simulink model "Peltier_OpenLoop_Simulink_Controller"  (R2018a)
settings: Solver=ode3  StartTime=0.0  StopTime=100  FixedStep=1/1000  RelTol=1e-3  EnableMultiTasking=on
libraries: simulink x1
settings Model: Creator=g.reynosomeza  LastModifiedBy=Pichau
settings DataIOCC: LimitDataPoints=on  SaveFormat=Array
settings OptimizationCC: LifeSpan=inf
settings DebuggingCC: AlgebraicLoopMsg=none  ArtificialAlgebraicLoopMsg=none  SolverPrmCheckMsg=warning  SFUnexpectedBacktrackingDiag=warning  SFNoUnconditionalDefaultTransitionDiag=warning  SFExecutionAtInitializationDiag=none
settings HardwareCC: ProdBitPerPointer=32  ProdBitPerSizeT=32  ProdBitPerPtrDiffT=32  ProdLargestAtomicFloat=None  ProdIntDivRoundTo=Undefined  ProdEndianess=Unspecified  ProdWordSize=32  ProdHWDeviceType=32-bit Generic
settings ModelReferenceCC: PropagateSignalLabelsOutOfModel=off
settings CodeAppCC: StateflowObjectComments=on
settings GRTTargetCC: TargetLangStandard=C89/C90 (ANSI)  GeneratePreprocessorConditionals=Disable all
settings ConfigComp: CovMetricSettings=dw  CovHtmlReporting=on  CovSaveCumulativeToWorkspaceVar=on  CovSaveSingleToWorkspaceVar=on  CovExternalEMLEnable=off  CovSFcnEnable=off

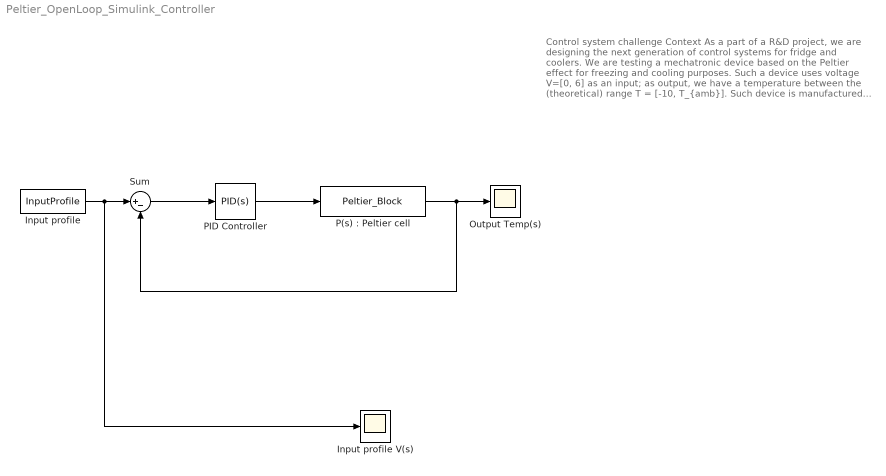
== system Peltier_OpenLoop_Simulink_Controller ==
  note: Control system challenge
      |
      | Context
      |
      | As a part of a R&D project, we are designing the next generation
      | of control systems for fridge and coolers. We are testing a mechatronic
      | device based on the Peltier effect for freezing and cooling purposes.
      | Such a device uses voltage V=[0, 6] as an input; as output, we have a
      | temperature between the (theoretical) range T = [-10, T_{amb}].
      |
      | Such device is manufactured in mass, and therefore, some differences
      | regarding physical properties are expected. We have a preliminary step-test
      | in order to appreciate the non-linear dynamic of the process.
      |
      | Task to perform
      |
      | It is desired to tune a controller, for the nominal process and robust enough
      | to handle the expected differences in its physical properties.
      |
      | 1) Controller performance will be evaluated with the IAE and TV indexes.
      | 2) Such controller must have a better performance when compared with a
      | controller adjusted with the Ziegler Nichols method. Otherwise, it will not
      | be considered as a control solution.
      |
      | Methodology
      |
      | 1) Control students will have access to a nominal process in Simulink. This mean
      | that we are expecting some differences regarding the dynamic behaviour in the
      | competition process.
      | 2) A temperature profile will be used for evaluation purposes.
      | Control students have a maximum of 2 tests with the competition model.
      | 3) Each controller will be ranked according to its dominance level, relative to
      | all solutions. Controller within the same dominance level will be ranked
      | according the TOPSIS criteria.
  Input profile : FromWorkspace  VariableName=InputProfile  SampleTime=0
  Input profile V(s) : Scope
  Output Temp(s) : Scope
  "P(s) : Peltier cell" : S-Function  FunctionName=Peltier_Block  SFunctionDeploymentMode=off  EnableBusSupport=off
  PID Controller : simulink/Continuous/PID Controller  Controller=PID  TimeDomain=Continuous-time  SampleTime=-1  IntegratorMethod=Forward Euler  FilterMethod=Forward Euler  Form=Parallel  UseFilter=on  ControllerParametersSource=internal  P=1  I=1  D=0  N=100  InitialConditionSource=internal  InitialConditionForIntegrator=0  InitialConditionForFilter=0  ExternalReset=none  LimitOutput=off  UpperSaturationLimit=inf  LowerSaturationLimit=-inf  LinearizeAsGain=on  AntiWindupMode=none  Kb=1  TrackingMode=off  Kt=1  PParamMin=[]  PParamMax=[]  IParamMin=[]  IParamMax=[]  DParamMin=[]  DParamMax=[]  NParamMin=[]  NParamMax=[]  KbParamMin=[]  KbParamMax=[]  KtParamMin=[]  KtParamMax=[]  POutMin=[]  POutMax=[]  IOutMin=[]  IOutMax=[]  DOutMin=[]  DOutMax=[]  NOutMin=[]  NOutMax=[]  KbOutMin=[]  KbOutMax=[]  KtOutMin=[]  KtOutMax=[]  IntegratorOutMin=[]  IntegratorOutMax=[]  FilterOutMin=[]  FilterOutMax=[]  SumOutMin=[]  SumOutMax=[]  SumI1OutMin=[]  SumI1OutMax=[]  SumI2OutMin=[]  SumI2OutMax=[]  SumI3OutMin=[]  SumI3OutMax=[]  SumDOutMin=[]  SumDOutMax=[]  SaturationOutMin=[]  SaturationOutMax=[]  IntegratorContinuousStateAttributes=''  IntegratorStateMustResolveToSignalObject=off  IntegratorRTWStateStorageClass=Auto  FilterContinuousStateAttributes=''  FilterStateMustResolveToSignalObject=off  FilterRTWStateStorageClass=Auto  DifferentiatorICPrevScaledInput=0  DifferentiatorOutMin=[]  DifferentiatorOutMax=[]  FilterDiffOutCoefMin=[]  FilterDiffOutCoefMax=[]  SumDenOutMin=[]  SumDenOutMax=[]  SumNumOutMin=[]  SumNumOutMax=[]  ReciprocalOutMin=[]  ReciprocalOutMax=[]  DivideOutMin=[]  DivideOutMax=[]  TunerSelectOption=Transfer Function Based (PID Tuner App)
  Sum : Sum  Inputs=|+-
  wires:
  "P(s) : Peltier cell"/1 -> Sum/2, Output Temp(s)/1
  Input profile/1 -> Sum/1, Input profile V(s)/1
  Sum/1 -> PID Controller/1
  PID Controller/1 -> "P(s) : Peltier cell"/1
